simulink library "GESMux"  (R2016b)
settings: Solver=VariableStepAuto  StartTime=0.0  StopTime=10.0  RelTol=1e-3
settings Model: Creator=MARCH  LastModifiedBy=MARCH

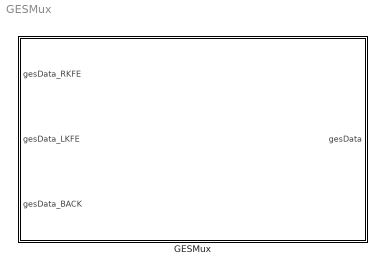
== system GESMux ==
  GESMux : Subsystem

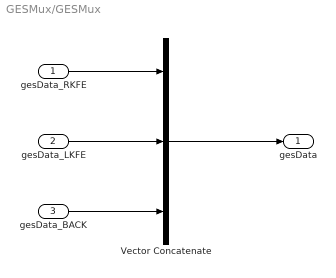
== system GESMux/GESMux ==
  gesData_RKFE : Inport
  gesData_LKFE : Inport  Port=2
  gesData_BACK : Inport  Port=3
  Vector Concatenate : Concatenate  NumInputs=3
  gesData : Outport
  wires:
  Vector Concatenate/1 -> gesData/1
  gesData_RKFE/1 -> Vector Concatenate/1
  gesData_LKFE/1 -> Vector Concatenate/2
  gesData_BACK/1 -> Vector Concatenate/3
